simulink model "untitled"  (R2019a)
settings: Solver=VariableStepAuto  StartTime=0.0  StopTime=10.0  RelTol=1e-3
settings Model: Creator=Qais  LastModifiedBy=Qais

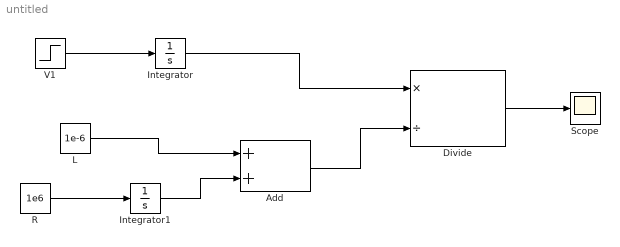
== system untitled ==
  "Add " : Sum
  "Divide " : Product  Inputs=*/
  "Integrator " : Integrator
  "Integrator1 " : Integrator
  L : Constant  Value=1e-6
  R : Constant  Value=1e6
  "Scope " : Scope
  V1 : Step  SampleTime=0
  wires:
  L/1 -> "Add "/1
  "Integrator1 "/1 -> "Add "/2
  R/1 -> "Integrator1 "/1
  V1/1 -> "Integrator "/1
  "Add "/1 -> "Divide "/2
  "Integrator "/1 -> "Divide "/1
  "Divide "/1 -> "Scope "/1
